simulink library "OmegaError"  (R2014b)
settings: Solver=ode45  StartTime=0.0  StopTime=10.0  RelTol=1e-3
settings Model: Creator=Hp  LastModifiedBy=Hp

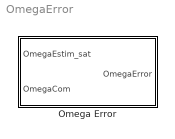
== system OmegaError ==
  Omega Error : Subsystem

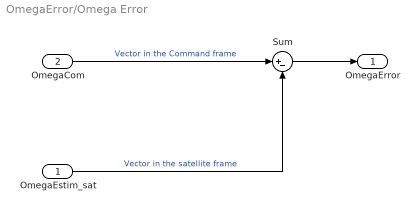
== system OmegaError/Omega Error ==
  OmegaEstim_sat : Inport
  OmegaCom : Inport  Port=2
  Sum : Sum  Inputs=|+-
  OmegaError : Outport
  wires:
  OmegaEstim_sat/1 -> Sum/2  "Vector in the satellite frame"
  OmegaCom/1 -> Sum/1  "Vector in the Command frame"
  Sum/1 -> OmegaError/1
